simulink model "StateMachine"  (R2021b)
settings: Solver=FixedStepDiscrete  StartTime=0.0  StopTime=20  FixedStep=0.001  RelTol=1e-3  EnableMultiTasking=on
settings Model: Creator=samwarner  LastModifiedBy=samwarner
settings SolverCC: ConcurrentTasks=on  AlgebraicLoopSolver=TrustRegion  AutoInsertRateTranBlk=on
settings DataIOCC: SaveFinalState=on  SaveState=on  DSMLogging=off  InspectSignalLogs=on
settings OptimizationCC: LifeSpan=inf
settings DebuggingCC: SFUnexpectedBacktrackingDiag=warning  SFNoUnconditionalDefaultTransitionDiag=warning  SFExecutionAtInitializationDiag=none  ArithmeticOperatorsInVariantConditions=warning
settings SFSimCC: SimUseLocalCustomCode=off  CustomCodeUndefinedFunction=UseInterfaceOnly
settings RTWCC: RTWUseLocalCustomCode=off
settings CodeAppCC: StateflowObjectComments=on
settings GRTTargetCC: TargetLangStandard=C89/C90 (ANSI)
settings ConfigComp: CovMetricSettings=dw  CovSaveCumulativeToWorkspaceVar=on  CovSaveSingleToWorkspaceVar=on  CovExternalEMLEnable=off

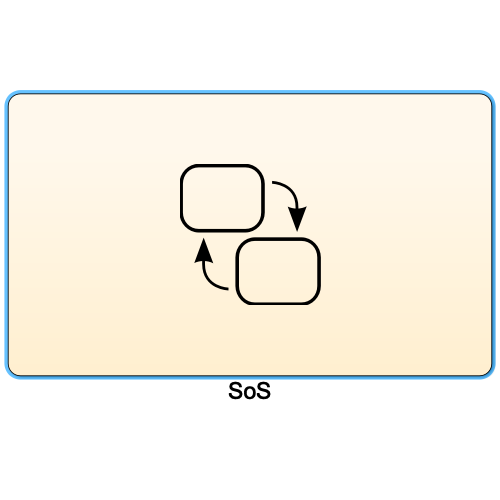
[thumbnail: Simulink's stored preview of the top-level diagram]
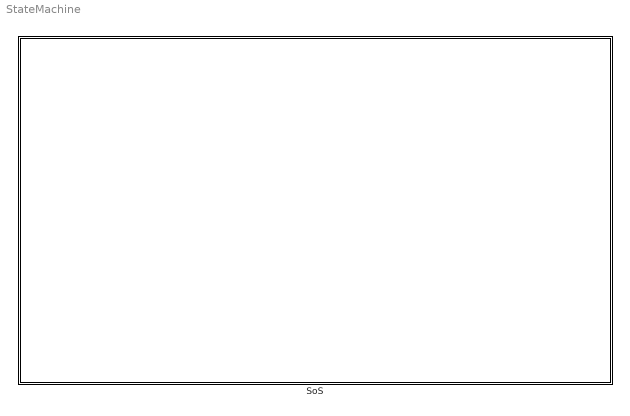
== system StateMachine ==
  SoS : Stateflow chart  TreatAsAtomicUnit=on

== stateflow chart StateMachine/SoS ==
  note: fundementals of Host Complete. Next Steps: (1)Convert Transittions to Local data, not Events. (2) add WILL. (3) add TCP unreliablility
  state SparkplugServer [parallel]
    settings: executionOrder=1
    state Connection1 [parallel]
      settings: executionOrder=1
      state Wait
        en:
        TcpConnected = 0;
        on after(1,sec):
        if TcpConnected ==0
        send(TCP_ESTABLISHED, ScadaHost);
        TcpConnected =1;
        end
      state Connect
        en:
        send(CONNACK, ScadaHost);
        send(Acked, SparkplugServer.Connection1);
      state Connected
        state Idle [parallel]
          settings: executionOrder=1
        state Publisher [parallel]
          on after(1,sec):
          send(PUBACK, ScadaHost);
          send(PUBACK, SparkplugServer.Connection1);
          settings: executionOrder=2
        state Subscribee [parallel]
          on after(1, sec):
          send(SUBACK, ScadaHost);
          send(SUBACK, SparkplugServer.Connection1);
          settings: executionOrder=3
        (default) -> SparkplugServer.Connection1.Connected.Idle
        SparkplugServer.Connection1.Connected.Idle -> SparkplugServer.Connection1.Connected.Publisher [order 1] : PUBLISH
        SparkplugServer.Connection1.Connected.Idle -> SparkplugServer.Connection1.Connected.Subscribee [order 2] : SUBSCRIBE
        SparkplugServer.Connection1.Connected.Publisher -> SparkplugServer.Connection1.Connected.Idle : PUBACK
        SparkplugServer.Connection1.Connected.Subscribee -> SparkplugServer.Connection1.Connected.Idle : SUBACK
      (default) -> SparkplugServer.Connection1.Wait
      SparkplugServer.Connection1.Wait -> SparkplugServer.Connection1.Connect : CONNECT
      SparkplugServer.Connection1.Connect -> SparkplugServer.Connection1.Connected : Acked
    state Connection2 [parallel]
      settings: executionOrder=2
      state Wait
        en:
        TcpConnection2Connected = 0;
        on after(1,sec):
        if TcpConnection2Connected ==0
        send(TCP_ESTABLISHED, EoN_Node);
        TcpConnection2Connected =1;
        end
      state Connect
        en:
        send(CONNACK, EoN_Node);
        send(Acked, SparkplugServer.Connection2);
      state Connected
        state Idle [parallel]
          settings: executionOrder=3
        state Publisher [parallel]
          on after(1,sec):
          send(PUBACK, EoN_Node);
          send(PUBACK, SparkplugServer.Connection2);
          settings: executionOrder=2
        state Subscribee [parallel]
          on after(1, sec):
          send(SUBACK, EoN_Node);
          send(SUBACK, SparkplugServer.Connection2);
          settings: executionOrder=1
        (default) -> SparkplugServer.Connection2.Connected.Idle
        SparkplugServer.Connection2.Connected.Idle -> SparkplugServer.Connection2.Connected.Publisher [order 1] : PUBLISH
        SparkplugServer.Connection2.Connected.Idle -> SparkplugServer.Connection2.Connected.Subscribee [order 2] : SUBSCRIBE
        SparkplugServer.Connection2.Connected.Publisher -> SparkplugServer.Connection2.Connected.Idle : PUBACK
        SparkplugServer.Connection2.Connected.Subscribee -> SparkplugServer.Connection2.Connected.Idle : SUBACK
      (default) -> SparkplugServer.Connection2.Wait
      SparkplugServer.Connection2.Wait -> SparkplugServer.Connection2.Connect : CONNECT
      SparkplugServer.Connection2.Connect -> SparkplugServer.Connection2.Connected : Acked
  state EoN_Node [parallel]
    settings: executionOrder=3
    state Initialization
      en:
      EoNConversationEstablished = 0;
      EoNSubscribeConversation = 0;
      EoNPublishConversation =0;
    state Wait
      en:
      send(CONNECT, SparkplugServer.Connection2);
    state Connected
      state Idle [parallel]
        du:
        if EoNConversationEstablished ==0
        send(EstablishSTATE, EoN_Node.Connected.Idle);
        send(SubscribeEoN, EoN_Node.Connected.Idle);
        EoNConversationEstablished =1;
        end
        settings: executionOrder=1
      state EstablishPub [parallel]
        on after(1, sec):
        if EoNPublishConversation == 0
        send(PUBLISH, SparkplugServer.Connection2);
        end
        EoNPublishConversation =1;
        settings: executionOrder=2
      state EstablishSub [parallel]
        on after(1, sec):
        if (EoNSubscribeConversation == 0)
        send(SUBSCRIBE, SparkplugServer.Connection2);
        end
        EoNSubscribeConversation = 1;
        settings: executionOrder=3
      (default) -> EoN_Node.Connected.Idle
      EoN_Node.Connected.Idle -> EoN_Node.Connected.EstablishSub [order 1] : SubscribeEoN
      EoN_Node.Connected.Idle -> EoN_Node.Connected.EstablishPub [order 2] : EstablishSTATE
      EoN_Node.Connected.EstablishPub -> EoN_Node.Connected.Idle : PUBACK
      EoN_Node.Connected.EstablishSub -> EoN_Node.Connected.Idle : SUBACK
    (default) -> EoN_Node.Initialization
    EoN_Node.Initialization -> EoN_Node.Wait : TCP_ESTABLISHED
    EoN_Node.Wait -> EoN_Node.Connected : CONNACK
  state ScadaHost [parallel]
    settings: executionOrder=2
    state Initialization
      en:
      ConversationEstablished = 0;
      SubscribeConversation = 0;
      PublishConversation =0;
    state Wait
      en:
      send(CONNECT, SparkplugServer.Connection1);
    state Connected
      state Idle [parallel]
        du:
        if ConversationEstablished ==0
        send(EstablishSTATE, ScadaHost.Connected.Idle);
        send(SubscribeEoN, ScadaHost.Connected.Idle);
        ConversationEstablished =1;
        end
        settings: executionOrder=1
      state EstablishPub [parallel]
        on after(1, sec):
        if PublishConversation == 0
        send(PUBLISH, SparkplugServer.Connection1);
        end
        PublishConversation =1;
        settings: executionOrder=2
      state EstablishSub [parallel]
        on after(1, sec):
        if (SubscribeConversation == 0)
        send(SUBSCRIBE, SparkplugServer.Connection1);
        end
        SubscribeConversation = 1;
        settings: executionOrder=3
      (default) -> ScadaHost.Connected.Idle
      ScadaHost.Connected.Idle -> ScadaHost.Connected.EstablishSub [order 1] : SubscribeEoN
      ScadaHost.Connected.Idle -> ScadaHost.Connected.EstablishPub [order 2] : EstablishSTATE
      ScadaHost.Connected.EstablishPub -> ScadaHost.Connected.Idle : PUBACK
      ScadaHost.Connected.EstablishSub -> ScadaHost.Connected.Idle : SUBACK
    (default) -> ScadaHost.Initialization
    ScadaHost.Initialization -> ScadaHost.Wait : TCP_ESTABLISHED
    ScadaHost.Wait -> ScadaHost.Connected : CONNACK
  data: TcpConnected local; ConversationEstablished local; SubscribeConversation local; PublishConversation local; TcpConnection2Connected local; EoNConversationEstablished local; EoNSubscribeConversation local; EoNPublishConversation local
  events: SubscribeEoN local FUNCTION_CALL_EVENT; EstablishSTATE local FUNCTION_CALL_EVENT; PUBACK local FUNCTION_CALL_EVENT; CONNECT local FUNCTION_CALL_EVENT; CONNACK local FUNCTION_CALL_EVENT; TCP_ESTABLISHED local FUNCTION_CALL_EVENT; PUBLISH local FUNCTION_CALL_EVENT; SUBACK local FUNCTION_CALL_EVENT; SUBSCRIBE local FUNCTION_CALL_EVENT; Acked local FUNCTION_CALL_EVENT
